simulink library "sm_car_lib"  (R2023a)
settings: Solver=VariableStepAuto  StartTime=0.0  StopTime=10.0  RelTol=1e-3
undefined symbols (not defined in the file or in its folder): Brakes, clr_upr, hp_la_out, hp_ua_out, opc_upr, radius_upr, rhs_hp, Steer, Z
libraries: Scene_Utilities x11, Suspension_Utilities x11, Vehicle_Inputs x5, Body_Utilities x3, World_Config_Utilities x2, Tire_Delft x2, Body_Axle1 x1, Body_Axle2 x1, Body_Axle3 x1, Brakes_Axle2_HydraulicValves_Channel4 x1, Brakes_Axle3_HydraulicValves_Channel6 x1, Brakes_Axle1_PedalAbstract_Disc x1
Description:
  | Simscape Vehicle Templates Library
  | 
  | Copyright 2018-2024 The MathWorks, Inc.
settings Model: Creator=mwalker  LastModifiedBy=smiller
settings SolverCC: AlgebraicLoopSolver=TrustRegion
settings DataIOCC: ReturnWorkspaceOutputs=off
settings DebuggingCC: UnconnectedInputMsg=warning  UnconnectedOutputMsg=warning  UnconnectedLineMsg=warning  ArithmeticOperatorsInVariantConditions=warning
settings ModelReferenceCC: EnableRefExpFcnMdlSchedulingChecks=on
settings SFSimCC: SimUseLocalCustomCode=off  CustomCodeUndefinedFunction=UseInterfaceOnly
settings RTWCC: RTWUseLocalCustomCode=off

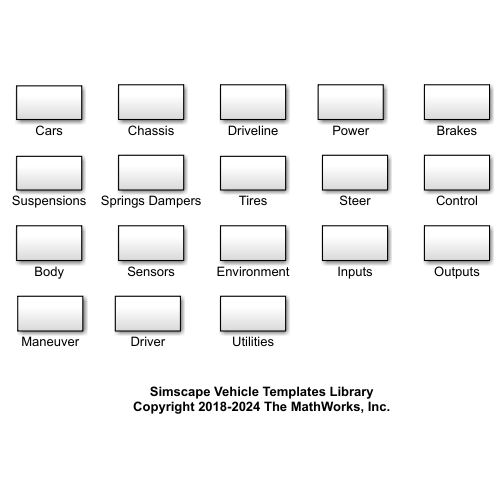
[thumbnail: Simulink's stored preview of the top-level diagram]
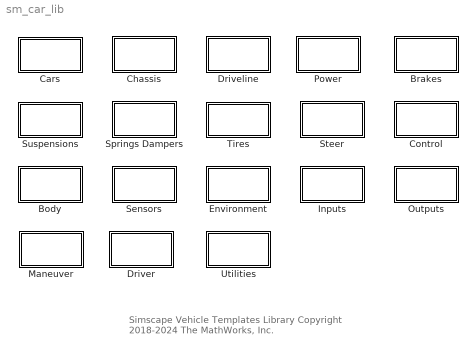
== system sm_car_lib ==
  note: Simscape Vehicle Templates Library
      | Copyright 2018-2024 The MathWorks, Inc.
  Body : Subsystem
  Brakes : Subsystem
  Cars : Subsystem
  Chassis : Subsystem
  Control : Subsystem
  Driveline : Subsystem
  Driver : Subsystem
  Environment : Subsystem
  Inputs : Subsystem
  Maneuver : Subsystem
  Outputs : Subsystem
  Power : Subsystem
  Sensors : Subsystem
  Springs Dampers : Subsystem
  Steer : Subsystem
  Suspensions : Subsystem
  Tires : Subsystem
  Utilities : Subsystem

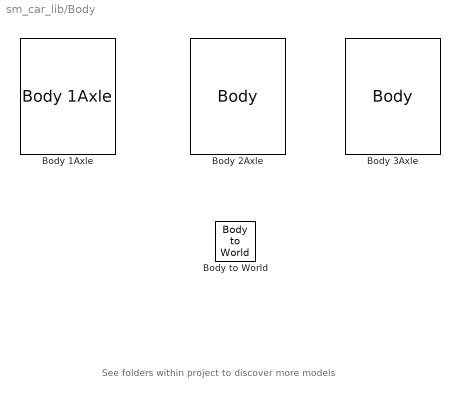
== system sm_car_lib/Body ==
  note: See folders within project to discover more models
  Body 1Axle : Body_Axle1/Body 1Axle  hp_mount_fa=Chassis.Body.sAxleF.Value  hp_mount_hitch=Chassis.Body.sAxleR.Value  hp_mount_power=Chassis.Body.sPower.Value  hp_chassis_cg=Chassis.Body.sCG.Value  chassis_mass=Chassis.Body.m.Value  chassis_inertia=Chassis.Body.J.Value  clr_chassis_hp_cg=Visual.hp.clr  opc_chassis_hp_cg=Visual.hp.opc  size_chassis_hp_cg=Visual.hp.rad  BodyGeometry=Chassis.Body.BodyGeometry
  Body 2Axle : Body_Axle2/Body  hp_mount_a1=Chassis.Body.sAxle1.Value  hp_mount_a2=Chassis.Body.sAxle2.Value  hp_mount_power=Vehicle.Chassis.Body.sPower.Value  hp_chassis_cg=Vehicle.Chassis.Body.sCG.Value  hp_mount_hitchf=Chassis.Body.sHitchF.Value  hp_mount_hitchr=Vehicle.Chassis.Body.sHitchR.Value  chassis_mass=Vehicle.Chassis.Body.m.Value  chassis_inertia=Vehicle.Chassis.Body.J.Value  clr_chassis_hp_cg=Visual.hp.clr  opc_chassis_hp_cg=Visual.hp.opc  size_chassis_hp_cg=Visual.hp.rad  BodyGeometry=Vehicle.Chassis.Body.BodyGeometry  Passenger=Vehicle.Chassis.Body.Passenger  BodyLoad=Body.BodyLoad
  Body 3Axle : Body_Axle3/Body  hp_mount_a1=Chassis.Body.sAxle1.Value  hp_mount_a2=Chassis.Body.sAxle2.Value  hp_mount_a3=Chassis.Body.sAxle3.Value  hp_mount_power=Vehicle.Chassis.Body.sPower.Value  hp_chassis_cg=Vehicle.Chassis.Body.sCG.Value  hp_mount_hitchf=Chassis.Body.sHitchF.Value  hp_mount_hitchr=Vehicle.Chassis.Body.sHitchR.Value  chassis_mass=Vehicle.Chassis.Body.m.Value  chassis_inertia=Vehicle.Chassis.Body.J.Value  clr_chassis_hp_cg=Visual.hp.clr  opc_chassis_hp_cg=Visual.hp.opc  size_chassis_hp_cg=Visual.hp.rad  BodyGeometry=Vehicle.Chassis.Body.BodyGeometry  Passenger=Vehicle.Chassis.Body.Passenger
  Body to World : Body_Utilities/Body to World  Init=Init.Chassis  SpecifyPosTarget=on

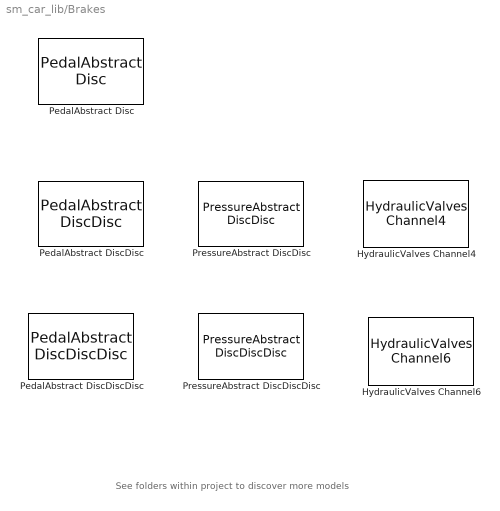
== system sm_car_lib/Brakes ==
  note: See folders within project to discover more models
  HydraulicValves Channel4 : Brakes_Axle2_HydraulicValves_Channel4/HydraulicValves Channel4  Tag=PublishSubsystem  VariantControl=HydraulicValves_Channel4  d_caliper_bore_a1=Brakes.Axle1.Caliper.lCylinderDiameter.Value  d_caliper_bore_a2=Brakes.Axle2.Caliper.lCylinderDiameter.Value  brk_pad_rad_a1=Brakes.Axle1.DiscAndPad.lMeanRadius.Value  brk_pad_rad_a2=Brakes.Axle2.DiscAndPad.lMeanRadius.Value  brk_cyl_bore_a1=Brakes.Axle1.Caliper.lCylinderDiameter.Value  brk_cyl_bore_a2=Brakes.Axle2.Caliper.lCylinderDiameter.Value  brk_n_pads_a1=Brakes.Axle1.DiscAndPad.NPads.Value  brk_n_pads_a2=Brakes.Axle2.DiscAndPad.NPads.Value  brk_mu_static_a1=Brakes.Axle1.DiscAndPad.rMuStatic.Value  brk_mu_static_a2=Brakes.Axle2.DiscAndPad.rMuStatic.Value  brk_mu_kin_a1=Brakes.Axle1.DiscAndPad.rMuKinetic.Value  brk_mu_kin_a2=Brakes.Axle2.DiscAndPad.rMuKinetic.Value  brk_trans_vel_a1=Brakes.Axle1.DiscAndPad.nTransition.Value  brk_trans_vel_a2=Brakes.Axle2.DiscAndPad.nTransition.Value  brk_visc_coef_a1=Brakes.Axle1.DiscAndPad.dViscous.Value  brk_visc_coef_a2=Brakes.Axle2.DiscAndPad.dViscous.Value  spr_rate=Brakes.Axle1.ValveApply.kSpring.Value  D=Brakes.Axle1.ValveApply.bDamper.Value  area_max_apply=Brakes.Axle1.ValveApply.AMax.Value  open_max_apply=Brakes.Axle1.ValveApply.xMax.Value  area_max_rel=Brakes.Axle1.ValveRelease.AMax.Value  open_max_rel=Brakes.Axle1.ValveRelease.xMax.Value  p_max_a1=Brakes.Axle1.Caliper.pMax.Value  p_max_a2=Brakes.Axle2.Caliper.pMax.Value  brkTs=Brakes.Axle1.ValveApply.fValveTime.Value
  HydraulicValves Channel6 : Brakes_Axle3_HydraulicValves_Channel6/HydraulicValves Channel6  Tag=PublishSubsystem  VariantControl=HydraulicValves_Channel6  d_caliper_bore_a1=Brakes.Axle1.Caliper.lCylinderDiameter.Value  d_caliper_bore_a2=Brakes.Axle2.Caliper.lCylinderDiameter.Value  d_caliper_bore_a3=Brakes.Axle3.Caliper.lCylinderDiameter.Value  brk_pad_rad_a1=Brakes.Axle1.DiscAndPad.lMeanRadius.Value  brk_pad_rad_a2=Brakes.Axle2.DiscAndPad.lMeanRadius.Value  brk_pad_rad_a3=Brakes.Axle3.DiscAndPad.lMeanRadius.Value  brk_cyl_bore_a1=Brakes.Axle1.Caliper.lCylinderDiameter.Value  brk_cyl_bore_a2=Brakes.Axle2.Caliper.lCylinderDiameter.Value  brk_cyl_bore_a3=Brakes.Axle3.Caliper.lCylinderDiameter.Value  brk_n_pads_a1=Brakes.Axle1.DiscAndPad.NPads.Value  brk_n_pads_a2=Brakes.Axle2.DiscAndPad.NPads.Value  brk_n_pads_a3=Brakes.Axle3.DiscAndPad.NPads.Value  brk_mu_static_a1=Brakes.Axle1.DiscAndPad.rMuStatic.Value  brk_mu_static_a2=Brakes.Axle2.DiscAndPad.rMuStatic.Value  brk_mu_static_a3=Brakes.Axle3.DiscAndPad.rMuStatic.Value  brk_mu_kin_a1=Brakes.Axle1.DiscAndPad.rMuKinetic.Value  brk_mu_kin_a2=Brakes.Axle2.DiscAndPad.rMuKinetic.Value  brk_mu_kin_a3=Brakes.Axle3.DiscAndPad.rMuKinetic.Value  brk_trans_vel_a1=Brakes.Axle1.DiscAndPad.nTransition.Value  brk_trans_vel_a2=Brakes.Axle2.DiscAndPad.nTransition.Value  brk_trans_vel_a3=Brakes.Axle3.DiscAndPad.nTransition.Value  brk_visc_coef_a1=Brakes.Axle1.DiscAndPad.dViscous.Value  brk_visc_coef_a2=Brakes.Axle2.DiscAndPad.dViscous.Value  brk_visc_coef_a3=Brakes.Axle3.DiscAndPad.dViscous.Value  spr_rate=Brakes.Axle1.ValveApply.kSpring.Value  D=Brakes.Axle1.ValveApply.bDamper.Value  area_max_apply=Brakes.Axle1.ValveApply.AMax.Value  open_max_apply=Brakes.Axle1.ValveApply.xMax.Value  area_max_rel=Brakes.Axle1.ValveRelease.AMax.Value  open_max_rel=Brakes.Axle1.ValveRelease.xMax.Value  p_max_a1=Brakes.Axle1.Caliper.pMax.Value  p_max_a2=Brakes.Axle2.Caliper.pMax.Value  p_max_a3=Brakes.Axle3.Caliper.pMax.Value  brkTs=Brakes.Axle1.ValveApply.fValveTime.Value
  PedalAbstract Disc : Brakes_Axle1_PedalAbstract_Disc/PedalAbstract Disc  Tag=PublishSubsystem  VariantControl=PedalAbstract_Disc  brk_pad_rad_a1=Brakes.Axle1.DiscAndPad.lMeanRadius.Value  brk_cyl_bore_a1=Brakes.Axle1.Caliper.lCylinderDiameter.Value  brk_n_pads_a1=Brakes.Axle1.DiscAndPad.NPads.Value  brk_mu_static_a1=Brakes.Axle1.DiscAndPad.rMuStatic.Value  brk_mu_kin_a1=Brakes.Axle1.DiscAndPad.rMuKinetic.Value  brk_trans_vel_a1=Brakes.Axle1.DiscAndPad.nTransition.Value  brk_visc_coef_a1=Brakes.Axle1.DiscAndPad.dViscous.Value  brk_max_p_a1=Brakes.Axle1.Caliper.pMax.Value  brk_filt_a1=1/Brakes.Axle1.Caliper.fActuatorCutoff.Value
  PedalAbstract DiscDisc : Brakes_Axle2_PedalAbstract_DiscDisc/PedalAbstract DiscDisc  Tag=PublishSubsystem  VariantControl=PedalAbstract_DiscDisc  brk_pad_rad_a1=Brakes.Axle1.DiscAndPad.lMeanRadius.Value  brk_pad_rad_a2=Brakes.Axle2.DiscAndPad.lMeanRadius.Value  brk_cyl_bore_a1=Brakes.Axle1.Caliper.lCylinderDiameter.Value  brk_cyl_bore_a2=Brakes.Axle2.Caliper.lCylinderDiameter.Value  brk_n_pads_a1=Brakes.Axle1.DiscAndPad.NPads.Value  brk_n_pads_a2=Brakes.Axle2.DiscAndPad.NPads.Value  brk_mu_static_a1=Brakes.Axle1.DiscAndPad.rMuStatic.Value  brk_mu_static_a2=Brakes.Axle2.DiscAndPad.rMuStatic.Value  brk_mu_kin_a1=Brakes.Axle1.DiscAndPad.rMuKinetic.Value  brk_mu_kin_a2=Brakes.Axle2.DiscAndPad.rMuKinetic.Value  brk_trans_vel_a1=Brakes.Axle1.DiscAndPad.nTransition.Value  brk_trans_vel_a2=Brakes.Axle2.DiscAndPad.nTransition.Value  brk_visc_coef_a1=Brakes.Axle1.DiscAndPad.dViscous.Value  brk_visc_coef_a2=Brakes.Axle2.DiscAndPad.dViscous.Value  brk_max_p_a1=Brakes.Axle1.Caliper.pMax.Value  brk_max_p_a2=Brakes.Axle2.Caliper.pMax.Value  brk_filt_a1=1/Brakes.Axle1.Caliper.fActuatorCutoff.Value  brk_filt_a2=1/Brakes.Axle2.Caliper.fActuatorCutoff.Value
  PedalAbstract DiscDiscDisc : Brakes_Axle3_PedalAbstract_DiscDiscDisc/PedalAbstract DiscDiscDisc  Tag=PublishSubsystem  VariantControl=PedalAbstract_DiscDiscDisc  brk_pad_rad_a1=Brakes.Axle1.DiscAndPad.lMeanRadius.Value  brk_pad_rad_a2=Brakes.Axle2.DiscAndPad.lMeanRadius.Value  brk_pad_rad_a3=Brakes.Axle3.DiscAndPad.lMeanRadius.Value  brk_cyl_bore_a1=Brakes.Axle1.Caliper.lCylinderDiameter.Value  brk_cyl_bore_a2=Brakes.Axle2.Caliper.lCylinderDiameter.Value  brk_cyl_bore_a3=Brakes.Axle3.Caliper.lCylinderDiameter.Value  brk_n_pads_a1=Brakes.Axle1.DiscAndPad.NPads.Value  brk_n_pads_a2=Brakes.Axle2.DiscAndPad.NPads.Value  brk_n_pads_a3=Brakes.Axle3.DiscAndPad.NPads.Value  brk_mu_static_a1=Brakes.Axle1.DiscAndPad.rMuStatic.Value  brk_mu_static_a2=Brakes.Axle2.DiscAndPad.rMuStatic.Value  brk_mu_static_a3=Brakes.Axle3.DiscAndPad.rMuStatic.Value  brk_mu_kin_a1=Brakes.Axle1.DiscAndPad.rMuKinetic.Value  brk_mu_kin_a2=Brakes.Axle2.DiscAndPad.rMuKinetic.Value  brk_mu_kin_a3=Brakes.Axle3.DiscAndPad.rMuKinetic.Value  brk_trans_vel_a1=Brakes.Axle1.DiscAndPad.nTransition.Value  brk_trans_vel_a2=Brakes.Axle2.DiscAndPad.nTransition.Value  brk_trans_vel_a3=Brakes.Axle3.DiscAndPad.nTransition.Value  brk_visc_coef_a1=Brakes.Axle1.DiscAndPad.dViscous.Value  brk_visc_coef_a2=Brakes.Axle2.DiscAndPad.dViscous.Value  brk_visc_coef_a3=Brakes.Axle3.DiscAndPad.dViscous.Value  brk_max_p_a1=Brakes.Axle1.Caliper.pMax.Value  brk_max_p_a2=Brakes.Axle2.Caliper.pMax.Value  brk_max_p_a3=Brakes.Axle3.Caliper.pMax.Value  brk_filt_a1=1/Brakes.Axle1.Caliper.fActuatorCutoff.Value  brk_filt_a2=1/Brakes.Axle2.Caliper.fActuatorCutoff.Value  brk_filt_a3=1/Brakes.Axle3.Caliper.fActuatorCutoff.Value
  PressureAbstract DiscDisc : Brakes_Axle2_PressureAbstract_DiscDisc/PressureAbstract DiscDisc  Tag=PublishSubsystem  VariantControl=PressureAbstract_DiscDisc  brk_pad_rad_a1=Brakes.Axle1.DiscAndPad.lMeanRadius.Value  brk_pad_rad_a2=Brakes.Axle2.DiscAndPad.lMeanRadius.Value  brk_cyl_bore_a1=Brakes.Axle1.Caliper.lCylinderDiameter.Value  brk_cyl_bore_a2=Brakes.Axle2.Caliper.lCylinderDiameter.Value  brk_n_pads_a1=Brakes.Axle1.DiscAndPad.NPads.Value  brk_n_pads_a2=Brakes.Axle2.DiscAndPad.NPads.Value  brk_mu_static_a1=Brakes.Axle1.DiscAndPad.rMuStatic.Value  brk_mu_static_a2=Brakes.Axle2.DiscAndPad.rMuStatic.Value  brk_mu_kin_a1=Brakes.Axle1.DiscAndPad.rMuKinetic.Value  brk_mu_kin_a2=Brakes.Axle2.DiscAndPad.rMuKinetic.Value  brk_trans_vel_a1=Brakes.Axle1.DiscAndPad.nTransition.Value  brk_trans_vel_a2=Brakes.Axle2.DiscAndPad.nTransition.Value  brk_visc_coef_a1=Brakes.Axle1.DiscAndPad.dViscous.Value  brk_visc_coef_a2=Brakes.Axle2.DiscAndPad.dViscous.Value  brk_filt_a1=1/Brakes.Axle1.Caliper.fActuatorCutoff.Value  brk_filt_a2=1/Brakes.Axle2.Caliper.fActuatorCutoff.Value
  PressureAbstract DiscDiscDisc : Brakes_Axle3_PressureAbstract_DiscDiscDisc/PressureAbstract DiscDiscDisc  Tag=PublishSubsystem  VariantControl=PressureAbstract_DiscDiscDisc  brk_pad_rad_a1=Brakes.Axle1.DiscAndPad.lMeanRadius.Value  brk_pad_rad_a2=Brakes.Axle2.DiscAndPad.lMeanRadius.Value  brk_pad_rad_a3=Brakes.Axle3.DiscAndPad.lMeanRadius.Value  brk_cyl_bore_a1=Brakes.Axle1.Caliper.lCylinderDiameter.Value  brk_cyl_bore_a2=Brakes.Axle2.Caliper.lCylinderDiameter.Value  brk_cyl_bore_a3=Brakes.Axle3.Caliper.lCylinderDiameter.Value  brk_n_pads_a1=Brakes.Axle1.DiscAndPad.NPads.Value  brk_n_pads_a2=Brakes.Axle2.DiscAndPad.NPads.Value  brk_n_pads_a3=Brakes.Axle3.DiscAndPad.NPads.Value  brk_mu_static_a1=Brakes.Axle1.DiscAndPad.rMuStatic.Value  brk_mu_static_a2=Brakes.Axle2.DiscAndPad.rMuStatic.Value  brk_mu_static_a3=Brakes.Axle3.DiscAndPad.rMuStatic.Value  brk_mu_kin_a1=Brakes.Axle1.DiscAndPad.rMuKinetic.Value  brk_mu_kin_a2=Brakes.Axle2.DiscAndPad.rMuKinetic.Value  brk_mu_kin_a3=Brakes.Axle3.DiscAndPad.rMuKinetic.Value  brk_trans_vel_a1=Brakes.Axle1.DiscAndPad.nTransition.Value  brk_trans_vel_a2=Brakes.Axle2.DiscAndPad.nTransition.Value  brk_trans_vel_a3=Brakes.Axle3.DiscAndPad.nTransition.Value  brk_visc_coef_a1=Brakes.Axle1.DiscAndPad.dViscous.Value  brk_visc_coef_a2=Brakes.Axle2.DiscAndPad.dViscous.Value  brk_visc_coef_a3=Brakes.Axle3.DiscAndPad.dViscous.Value  brk_filt_a1=1/Brakes.Axle1.Caliper.fActuatorCutoff.Value  brk_filt_a2=1/Brakes.Axle2.Caliper.fActuatorCutoff.Value  brk_filt_a3=1/Brakes.Axle3.Caliper.fActuatorCutoff.Value

== system sm_car_lib/Cars ==
  note: See folders within project to discover more models
  Vehicle Axle1 : Vehicle_Axle1/Vehicle 1Axle  Tag=PublishSubsystem  VariantControl=NS_Con  Vehicle=Trailer  Init=Init  veh_index=61
  Vehicle Axle2 : Vehicle_Axle2/Vehicle  Tag=PublishSubsystem  VariantControl=NS_Con  Vehicle=Vehicle  Init=Init  SpecifyPosTarget=on  veh_index=1  mask_image_name=sm_car_vehicle_hamba_IMAGE.png
  Vehicle Axle3 : Vehicle_Axle3/Vehicle  Tag=PublishSubsystem  VariantControl=NS_Con  Vehicle=Vehicle  Init=Init  veh_index=1  mask_image_name=sm_car_vehicle_hambalg_IMAGE.png

== system sm_car_lib/Chassis ==
  note: See folders within project to discover more models
  Chassis Axle1 : Chassis_Axle1/Chassis  Tag=PublishSubsystem  VariantControl=Chassis  Chassis=Vehicle.Chassis  Init=Init  veh_index=61
  Chassis Axle2 : Chassis_Axle2/Chassis  Tag=PublishSubsystem  VariantControl=Chassis  Chassis=Vehicle.Chassis  Init=Init  mask_image_name=sm_car_vehicle_chassis_custom_IMAGE.png  veh_index=1
  Chassis Axle3 : Chassis_Axle3/Chassis  Tag=PublishSubsystem  VariantControl=Chassis  Chassis=Vehicle.Chassis  Init=Init  mask_image_name=sm_car_vehicle_chassis_custom_IMAGE.png  veh_index=1

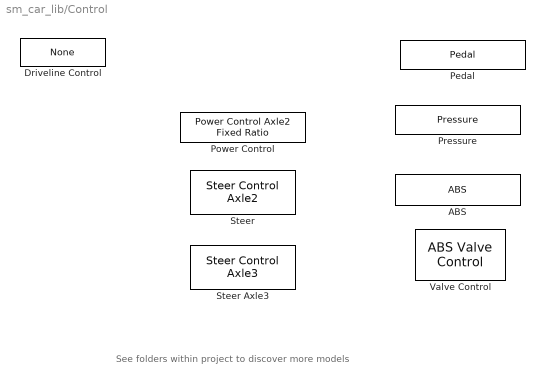
== system sm_car_lib/Control ==
  note: See folders within project to discover more models
  ABS : Brake_Control_ABS/ABS  VariantControl=ABS  abs_tire_radiusF=abs_tire_radiusF  abs_tire_radiusR=abs_tire_radiusR
  Driveline Control : Driveline_Control_Axle2_None/None  SystemSampleTime=-1  VariantActivationTime=update diagram  Latency=0  AutoFrameSizeCalculation=off
  Pedal : Brake_Control_Pedal/Pedal  SystemSampleTime=-1  VariantControl=Pedal  VariantActivationTime=update diagram  Latency=0  AutoFrameSizeCalculation=off
  Power Control : Power_Control_Axle2_FixedRatio/Power Control Axle2 Fixed Ratio  trq_max=1600  trq_ratio_front=1  trq_rate_up=300  trq_rate_down=-5000
  Pressure : Brake_Control_Pressure/Pressure  SystemSampleTime=-1  VariantControl=Pressure  VariantActivationTime=update diagram  Latency=0  AutoFrameSizeCalculation=off
  Steer : Steer_Control_Axle2/Steer Control Axle2  Steer=Control.Default.Steer
  Steer Axle3 : Steer_Control_Axle3/Steer Control Axle3  nSteerA2=Control.Default.steer_ratio_axle2  nSteerA3=Control.Default.steer_ratio_axle3
  Valve Control : Brake_Control_ABS_Valve/ABS Valve Control  SystemSampleTime=-1  VariantActivationTime=update diagram  Latency=0  AutoFrameSizeCalculation=off

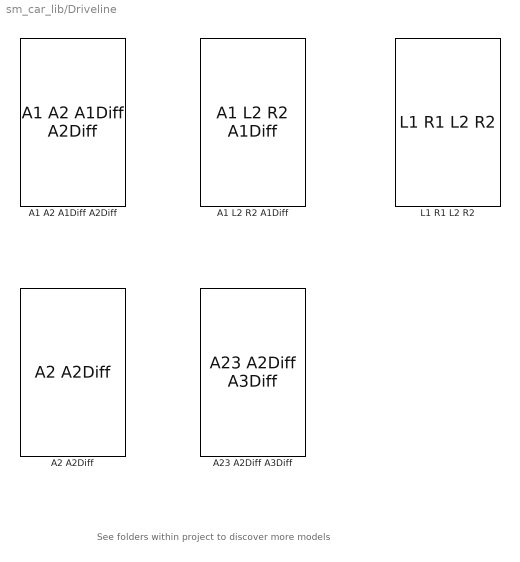
== system sm_car_lib/Driveline ==
  note: See folders within project to discover more models
  A1 A2 A1Diff A2Diff : Driveline_Axle2_A1_A2_A1Diff_A2Diff/A1 A2 A1Diff A2Diff  Tag=PublishSubsystem  VariantControl=A1_A2_A1Diff_A2Diff
  A1 L2 R2 A1Diff : Driveline_Axle2_A1_L2_R2_A1Diff/A1 L2 R2 A1Diff  Tag=PublishSubsystem  VariantControl=A1_L2_R2_A1Diff
  A2 A2Diff : Driveline_Axle3_A2_A2Diff/A2 A2Diff  Tag=PublishSubsystem  VariantControl=A2_A2Diff
  A23 A2Diff A3Diff : Driveline_Axle3_A23_A2Diff_A3Diff/A23 A2Diff A3Diff  Tag=PublishSubsystem  VariantControl=A23_A2Diff_A3Diff
  L1 R1 L2 R2 : Driveline_Axle2_L1_R1_L2_R2/L1 R1 L2 R2  Tag=PublishSubsystem  VariantControl=L1_R1_L2_R2

== system sm_car_lib/Driver ==
  note: See folders within project to discover more models
  Long Lat Stanley : Driver_Long_Lateral/Driver  Driver=Driver
  Open Loop : Driver_Open_Loop/Open Loop  Maneuver=Maneuver

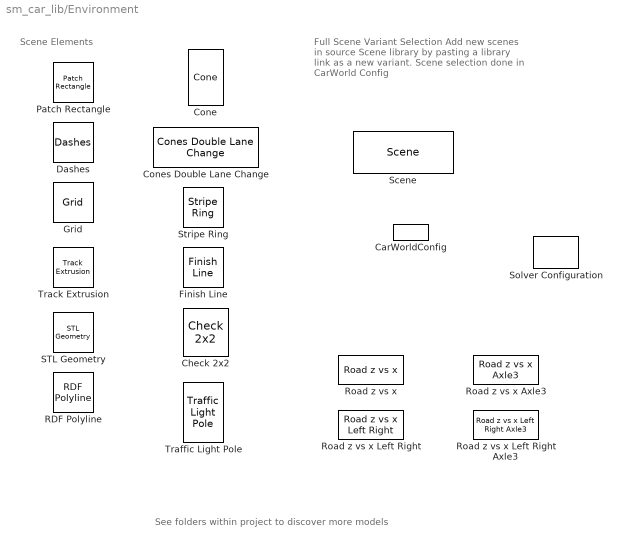
== system sm_car_lib/Environment ==
  note: Full Scene Variant Selection
      | Add new scenes in source
      | Scene library by pasting a library
      | link as a new variant.
      | Scene selection done
      | in CarWorld Config
  note: Scene Elements
  note: See folders within project to discover more models
  CarWorldConfig : World_Config_Utilities/CarWorldConfig  UseLocalSolver=off  LocalSolverChoice=Backward Euler  LocalSolverSampleTime=0.005  DoFixedCost=off  MaxNonlinIter=3  popup_scene=Plane Grid  popup_gravity=Constant  GravityVector=[0 0 -9.80665]
      settings: AttributesFormatString=|
      | %<popup_scene>
      | Local Solver: %<UseLocalSolver>
  Check 2x2 : Scene_Utilities/Check 2x2  square_lwh=[0.01 1 1]
  Cone : Scene_Utilities/Cone  height=1  baseThickness=0.1  baseWidth=0.6  coneBaseDiameter=0.4  coneTopDiameter=0.1  reflectiveStripHeight=0.5  coneColor=[1 0.6 0]  reflectiveStripColor=[0.75 0.75 0.75]
  Cones Double Lane Change : Scene_Utilities/Cones Double Lane Change  lane_width=3.3  lane_separation=4.1  start_lane_a=173.8  A1_to_A5=12.5  A_to_B_x=12.7  B1_to_B5=12.3  B_to_C_x=12.7  C1_to_C5=12  height=0.6  baseThickness=0.04  baseWidth=0.5  coneBaseDiameter=0.24  coneTopDiameter=0.06  reflectiveStripHeight=0.3  coneColor=[248 78 25]/255  reflectiveStripColor=[0.75 0.75 0.75]
  Dashes : Scene_Utilities/Dashes  dash_pitch=7.5  num_dashes=4  dash_l=3  dash_h=2  dash_w=0.15  thickness_base=4  dash_clr=[1 1 1]  dash_opc=1
  Finish Line : Scene_Utilities/Finish Line  post_h=6  post_r=0.5  line_w=18  post_clr=[0.8 0.0 0.2]  post_opc=1  offset_xyz=[0 0 0]  offset_yaw=0  offset_pitch=0  offset_roll=0
  Grid : Scene_Utilities/Grid  grid_x=400  grid_y=400  grid_z=0.02  grid_line_width=0.08  grid_num_sq_x=10  grid_num_sq_y=17  grid_clr=[1 1 1]  grid_opc=1
  Patch Rectangle : Scene_Utilities/Patch Rectangle  gp_l=400  gp_w=400  gp_h=0.01  gp_clr=[0.8000 0.8000 0.8000]  gp_opc=1
  RDF Polyline : Scene_Utilities/RDF Polyline  road_extr_data_L=RDF_Rough_Road.Road.extr_data_L  road_extr_data_R=RDF_Rough_Road.Road.extr_data_R  road_profile_sep=RDF_Rough_Road.Road.profile_separation  road_w=RDF_Rough_Road.Road.w  road_x=RDF_Rough_Road.Road.x  road_z=RDF_Rough_Road.Road.z  road_yaw=RDF_Rough_Road.Road.yaw  road_clr=RDF_Rough_Road.Road.clr  road_opc=RDF_Rough_Road.Road.opc
  Road z vs x Left Right : Surface_Profile_Axle2_zx_LR/Road z vs x Left Right  VariantControl=Variant  dist_x_l=flipud(Scene.RDF_Plateau.Road.extr_data_L(45:end,1))  height_z_l=flipud(Scene.RDF_Plateau.Road.extr_data_L(45:end,2))  dist_x_r=flipud(Scene.RDF_Plateau.Road.extr_data_R(45:end,1))  height_z_r=flipud(Scene.RDF_Plateau.Road.extr_data_R(45:end,2))
  Road z vs x Left Right Axle3 : Surface_Profile_Axle3_zx_LR/Road z vs x Left Right Axle3  VariantControl=Variant  dist_x_l=flipud(Scene.RDF_Plateau.Road.extr_data_L(45:end,1))  height_z_l=flipud(Scene.RDF_Plateau.Road.extr_data_L(45:end,2))  dist_x_r=flipud(Scene.RDF_Plateau.Road.extr_data_R(45:end,1))  height_z_r=flipud(Scene.RDF_Plateau.Road.extr_data_R(45:end,2))
  "Road z vs x " : Surface_Profile_Axle2_zx/Road z vs x   VariantControl=Variant  dist_x=flipud(Scene.RDF_Plateau.Road.extr_data_L(45:end,1))  height_z=flipud(Scene.RDF_Plateau.Road.extr_data_L(45:end,2))
  Road z vs x Axle3 : Surface_Profile_Axle3_zx/Road z vs x Axle3  VariantControl=Variant  dist_x=flipud(Scene.RDF_Plateau.Road.extr_data_L(45:end,1))  height_z=flipud(Scene.RDF_Plateau.Road.extr_data_L(45:end,2))
  STL Geometry : Scene_Utilities/STL Geometry  stl_file='Bar1_Default_sldprt.STL'  stl_units='m'  stl_clr=[0.8000 0.8000 0.8000]  stl_opc=1  stl_x=0  stl_y=0  stl_z=0  stl_yaw=0  stl_pitch=0  stl_roll=0
  Scene : Scene_Systems/Scene  SystemSampleTime=-1  LabelModeActiveChoice=Road_Two_Lane  VariantActivationTime=update diagram  Latency=0  AutoFrameSizeCalculation=off
      settings: AttributesFormatString=%<LabelModeActiveChoice>
  Solver Configuration : nesl_utility/Solver Configuration  PhysicalDomain=network_engine_domain  SubClassName=solver  LeftPortType=input  RightPortType=generic  Tones=[]  Harmonics=[]  SimulateNoise=off  Profile=off  UseLocalSampling=off  EnableSwitchedLinearOptims=on  FrequencyDomain=off  UseCCode=off  RelTol=0.001  AbsTol=1e-06  MinStep=1e-09  ToWorkspace=off  RevertToSquareIcSolve=off  NumHomotopyIterations=100  PhasorMode=off  PhasorModeNumHarmonics=1  IndexReductionMethod=DerivativeReplacement  DoDC=off  ResidualTolerance=1e-09  UseLocalSolver=on  LocalSolverChoice=NE_BACKWARD_EULER_ADVANCER  LocalSolverSampleTime=0.001  DoFixedCost=on  MaxNonlinIter=3  MaxModeIter=2  ComputeImpulses=off  ImpulseIterations=2  LinearAlgebra=auto  LinearAlgebraNumThread=0  EquationFormulation=NE_TIME_EF  DelaysMemoryBudget=1024  AutomaticFiltering=on  FilteringTimeConstant=0.001  PartitionStorageMethod=AS_NEEDED  PartitionMemoryBudget=1024  PartitionMethod=FAST
  Stripe Ring : Scene_Utilities/Stripe Ring  circ_d=circ_out.d  circ_a1=circ_out.ang1  circ_a2=circ_out.ang2  circ_w=circ_out.w  circ_h=circ_out.h  circ_clr=circ_out.clr  circ_opc=circ_out.opc
  Track Extrusion : Scene_Utilities/Track Extrusion  track_ctrline=[sin(0:0.1:(2*pi-0.1))' cos(0:0.1:(2*pi-0.1))' cos(0:0.1:(2*pi-0.1))']*10  track_w=2  track_h=0.1  track_x=0  track_y=0  track_z=0  track_yaw=0  track_clr=[0.8000 0.8000 0.8000]  track_opc=1
  Traffic Light Pole : Object_Traffic_Light/Traffic Light Pole  clr_tlp_housing=[0.5 0.5 0.5]  offset_tlp=[0 258 2]  orient_tlp=pi*1.1  pole_height_tlp=2

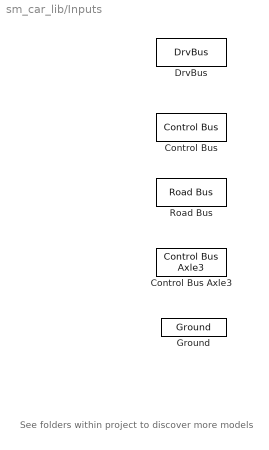
== system sm_car_lib/Inputs ==
  note: See folders within project to discover more models
  Control Bus : Vehicle_Inputs/Control Bus  SystemSampleTime=-1  VariantActivationTime=update diagram  Latency=0  AutoFrameSizeCalculation=off
  Control Bus Axle3 : Vehicle_Inputs/Control Bus Axle3  SystemSampleTime=-1  VariantActivationTime=update diagram  Latency=0  AutoFrameSizeCalculation=off
  DrvBus : Vehicle_Inputs/DrvBus  SystemSampleTime=-1  VariantActivationTime=update diagram  Latency=0  AutoFrameSizeCalculation=off
  Ground : Vehicle_Inputs/Ground  SystemSampleTime=-1  VariantActivationTime=update diagram  Latency=0  AutoFrameSizeCalculation=off
  Road Bus : Vehicle_Inputs/Road Bus  SystemSampleTime=-1  VariantActivationTime=update diagram  Latency=0  AutoFrameSizeCalculation=off

== system sm_car_lib/Maneuver ==
  note: See folders within project to discover more models
  Check : World_Config_Utilities/Check  stop_speed=0.1  start_check_time=5  max_speed=0.4  start_check_time_max_speed=20000  lat_dev_threshold=8  start_check_time_ld=10000  start_check_time_end_lap=10000
  Maneuver : Maneuver_Get_Pose/Maneuver  Maneuver=Maneuver  popup_window=No

== system sm_car_lib/Outputs ==
  note: See folders within project to discover more models
  Terminator : Terminator
  VehBus : Vehicle_Outputs/VehBus  SystemSampleTime=-1  VariantActivationTime=update diagram  Latency=0  AutoFrameSizeCalculation=off
  wires:
  VehBus/1 -> Terminator/1

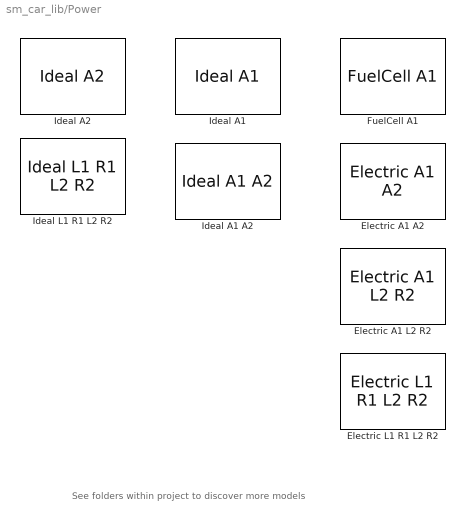
== system sm_car_lib/Power ==
  note: See folders within project to discover more models
  Electric A1 A2 : Power_Shaft2_Electric_A1_A2/Electric A1 A2  VariantControl=Electric_A1_A2  Power=Powertrain.Power
  Electric A1 L2 R2 : Power_Shaft3_Electric_A1_L2_R2/Electric A1 L2 R2  VariantControl=Electric_A1_L2_R2  Power=Powertrain.Power
  Electric L1 R1 L2 R2 : Power_Shaft4_Electric_L1_R1_L2_R2/Electric L1 R1 L2 R2  VariantControl=Electric_L1_R1_L2_R2  Power=Powertrain.Power
  FuelCell A1 : Power_Shaft1_FuelCell_A1/FuelCell A1  VariantControl=FuelCell_A1  Power=Powertrain.Power
  Ideal A1 : Power_Shaft1_Ideal_A1/Ideal A1  VariantControl=Ideal_A1  motor_ts_f=Power.ActuatorCutoffA1.Value
  Ideal A1 A2 : Power_Shaft2_Ideal_A1_A2/Ideal A1 A2  VariantControl=Ideal_A1_A2  motor_ts_a1=Power.ActuatorCutoffA1.Value  motor_ts_a2=Power.ActuatorCutoffA2.Value
  Ideal A2 : Power_Shaft1_Ideal_A2/Ideal A2  VariantControl=Ideal_A2  motor_ts_f=Power.ActuatorCutoffA2.Value
  Ideal L1 R1 L2 R2 : Power_Shaft4_Ideal_L1_R1_L2_R2/Ideal L1 R1 L2 R2  VariantControl=Ideal_L1_R1_L2_R2  motor_ts_l1=100  motor_ts_r1=100  motor_ts_l2=100  motor_ts_r2=100

== system sm_car_lib/Sensors ==
  note: See folders within project to discover more models
  Body Sensor : Body_Utilities/Body Sensor  offset_body_sensor=Vehicle.Chassis.Body.sCG.Value
  Body Sensor Empty : Body_Utilities/Body Sensor Empty  offset_body_sensor=Vehicle.Chassis.Body.sCG.Value

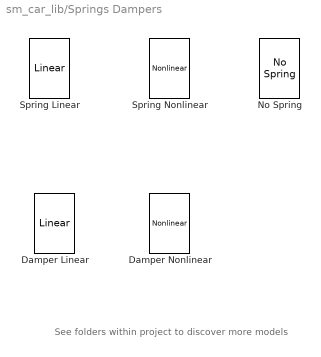
== system sm_car_lib/Springs Dampers ==
  note: See folders within project to discover more models
  Damper Linear : Damper_Linear/Linear  VariantControl=Linear  dam_b=Damper.Damping.d.Value  hp_dpr_top=Damper.Damping.sTop.Value  hp_dpr_bot=Damper.Damping.sBottom.Value  bs_lim_upper=Damper.Endstop.xMax.Value  bs_lim_lower=Damper.Endstop.xMin.Value  bs_k_upper=Damper.Endstop.KxMax.Value  bs_k_lower=Damper.Endstop.KxMin.Value  bs_b_upper=Damper.Endstop.dxMax.Value  bs_b_lower=Damper.Endstop.dxMin.Value  bs_region=Damper.Endstop.xTransition.Value
  Damper Nonlinear : Damper_Nonlinear/Nonlinear  VariantControl=Nonlinear  velocity_vector=Damper.Damping.vDamper.Value  force_vector=Damper.Damping.fDamper.Value  hp_dpr_top=Damper.Damping.sTop.Value  hp_dpr_bot=Damper.Damping.sBottom.Value  bs_lim_upper=Damper.Endstop.xMax.Value  bs_lim_lower=Damper.Endstop.xMin.Value  bs_k_upper=Damper.Endstop.KxMax.Value  bs_k_lower=Damper.Endstop.KxMin.Value  bs_b_upper=Damper.Endstop.dxMax.Value  bs_b_lower=Damper.Endstop.dxMin.Value  bs_region=Damper.Endstop.xTransition.Value
  No Spring : Spring_None/No Spring  VariantControl=No_Spring
  Spring Linear : Spring_Linear/Linear  VariantControl=Linear  spr_def0=Spring.xPreload.Value  spr_k=Spring.K.Value  spr_hp_top=Spring.sTop.Value  spr_hp_bot=Spring.sBottom.Value
  Spring Nonlinear : Spring_Nonlinear/Nonlinear  VariantControl=Nonlinear  spr_def0=Spring.xPreload.Value  deformation_vector=Spring.xSpring.Value  force_vector=Spring.fSpring.Value  spr_hp_top=Spring.sTop.Value  spr_hp_bot=Spring.sBottom.Value

== system sm_car_lib/Steer ==
  note: See folders within project to discover more models
  Rack : Steer_Rack_Only/Rack  Tag=PublishSubsystem  VariantControl=Rack  hp_mt_rack=Steer.Rack.sMount.Value  hp_out_rack=Steer.Rack.sOutboard.Value  rack_mass=Steer.Rack.m.Value  whl2rack_whlangle=Steer.Ratio_Table.aWheel.Value  whl2rack_rackdisp=Steer.Ratio_Table.xRack.Value  whl2rack_filter=1/Steer.Rack.fActuatorCutoff.Value  clr_rack=Visual.SteeringRack.clr  opc_rack=Visual.part.opc  radius_rack=Visual.SteeringRack.rad  clr_connhp=Visual.hp.clr  opc_connhp=Visual.hp.opc  size_connhp=Visual.hp.rad
  Rack Wheel : Steer_Rack_Wheel/Rack Wheel  Tag=PublishSubsystem  VariantControl=RackWheel  hp_wheel=Steer.Wheel.sMount.Value  wheel_axis_incl=Steer.Wheel.aAxis.Value  hp_mt_rack=Steer.Rack.sMount.Value  hp_out_rack=Steer.Rack.sOutboard.Value  Wheel=Steer.Wheel  rack_mass=Steer.Rack.m.Value  whl2rack_whlangle=Steer.Ratio_Table.aWheel.Value  whl2rack_rackdisp=Steer.Ratio_Table.xRack.Value  whl2rack_filter=1/Steer.Rack.fActuatorCutoff.Value  clr_rack=Visual.SteeringRack.clr  opc_rack=Visual.part.opc  radius_rack=Visual.SteeringRack.rad  clr_connhp=Visual.hp.clr  opc_connhp=Visual.hp.opc  size_connhp=Visual.hp.rad  clr_wheel=Visual.SteeringWheel.clr  opc_wheel=Visual.part.opc  DriverHuman=Steer.DriverHuman
  Wheel Driven Rack 1UJoint : Steer_Rack_WheelDrivenRack1UJoint/Wheel Driven Rack 1UJoint  Tag=PublishSubsystem  VariantControl=WheelDrivenRack1UJoint  hp_wheel=Steer.Wheel.sMount.Value  wheel_axis_incl=Steer.Wheel.aAxis.Value  hp_mt_rack=Steer.Rack.sMount.Value  hp_out_rack=Steer.Rack.sOutboard.Value  hp_pinion=Steer.Pinion.sMount.Value  Wheel=Steer.Wheel  len_sha_u=Steer.Shaft_Upper.xLength.Value  sha_u_mass=Steer.Shaft_Upper.m.Value  sha_l_mass=Steer.Shaft_Lower.m.Value  rad_pinion=Steer.Pinion.xRad.Value  pinion_mass=Steer.Pinion.m.Value  rack_mass=Steer.Rack.m.Value  whl2steer_filter=1/Steer.Rack.fActuatorCutoff.Value  clr_rack=Visual.SteeringRack.clr  opc_rack=Visual.part.opc  radius_rack=Visual.SteeringRack.rad  clr_shaft=Visual.SteeringShafts.clr  opc_shaft=Visual.part.opc  size_shaft=Visual.SteeringShafts.rad  clr_pinion=Visual.SteeringPinion.clr  opc_pinion=Visual.part.opc  len_pinion=Visual.SteeringPinion.len  clr_connhp=Visual.hp.clr  opc_connhp=Visual.hp.opc  size_connhp=Visual.hp.rad  clr_wheel=Visual.SteeringWheel.clr  opc_wheel=Visual.part.opc  DriverHuman=Steer.DriverHuman

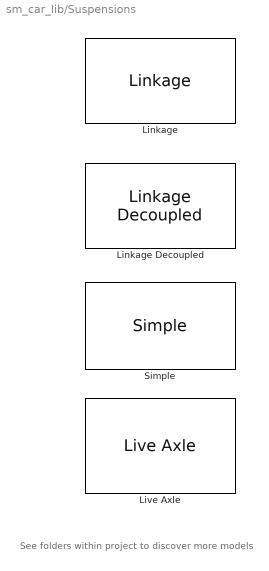
== system sm_car_lib/Suspensions ==
  note: See folders within project to discover more models
  Linkage : Suspension_Linkage/Linkage  VariantControl=Linkage
  Linkage Decoupled : Suspension_Linkage_Decoupled/Linkage Decoupled  VariantControl=Decoupled
  Live Axle : Suspension/Suspension and Steering/Live Axle  VariantControl=LiveAxle  LiveAxle=Susp.LiveAxle
  Simple : Susp_DOF15/Simple  VariantControl=Simple

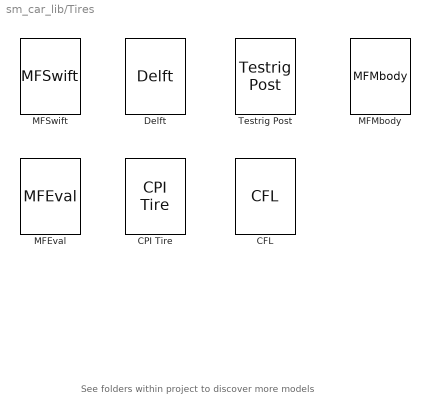
== system sm_car_lib/Tires ==
  note: See folders within project to discover more models
  CFL : Tire_CFL/CFL  VariantControl=CFL  popup_leftRight=Right  tire_radius=Tire.tire_radius.Value  rim_radius=Tire.rim_radius.Value  tire_width=Tire.tire_width.Value  rim_width=Tire.rim_width.Value  tyre_mass=Tire.tire_mass.Value  rim_mass=Tire.rim_mass.Value  tire_inertia=Tire.tire_J.Value  rim_inertia=Tire.rim_J.Value  plane_l=Tire.plane.l.Value  plane_w=Tire.plane.w.Value  k_contact=Tire.k.Value  b_contact=Tire.b.Value  mu_kinetic=Tire.mu_k.Value  mu_static=Tire.mu_s.Value  v_thr=Tire.v_thr.Value  TireBody=Tire.TireBody  clr_tyre_cfl=Visual.Tire.clr  opc_tyre_cfl=Visual.Tire.opc  clr_rim_cfl=Visual.Rim.clr  opc_rim_cfl=Visual.Rim.opc
  CPI Tire : Tire_Delft/CPI Tire  VariantControl=CPI  idtyre=0
  Delft : Tire_Delft/Delft  VariantControl=Delft  idtyre=tir_index  rim_inertia=Tire.mjRim.Value  tir_name=Tire.tirFile.Value  rdf_name=Tire.roadFile.Value  tire_side_mode=(2xxx) right  tire_contact=Tire.Contact.Value  tire_dynamics=Tire.Dynamics.Value  tire_slip=Tire.Slip.Value  TireBody=Tire.TireBody  popup_leftRight=Right  clr_tyre=Visual.Tire.clr  opc_tyre=Visual.Tire.opc  clr_rim=Visual.Rim.clr  opc_rim=Visual.Rim.opc
  MFEval : Tire_MFEval/MFEval  VariantControl=MFEval  tir_file=Tire.tirFile.Value  tir_side=2 right  tir_dynamics=Tire.Dynamics.Value  tir_mode=Tire.Slip.Value  TireBody=Tire.TireBody  popup_leftRight=Right  clr_tyre=Visual.Tire.clr  opc_tyre=Visual.Tire.opc  clr_rim=Visual.Rim.clr  opc_rim=Visual.Rim.opc
  MFMbody : Tire_MFMbody/MFMbody  VariantControl=MFMbody  tir_file=Tire.tirFile.Value  tire_side=Right  TireBody=Tire.TireBody  fcontactpatch=Tire.fContactPoint.Value  road_file=Tire.roadFile.Value  popup_leftRight=Right  clr_tyre=Visual.Tire.clr  opc_tyre=Visual.Tire.opc  clr_rim=Visual.Rim.clr  opc_rim=Visual.Rim.opc
  MFSwift : Tire_MFSwift/MFSwift  VariantControl=MFSwift  idtyre=tir_index  rim_inertia=Tire.mjRim.Value  tir_name=Tire.tirFile.Value  rdf_name=Tire.roadFile.Value  tire_side_mode=(x2xxx) right  tire_contact=Tire.Contact.Value  tire_dynamics=Tire.Dynamics.Value  tire_slip=Tire.Slip.Value  solver_enable=Tire.InternalSolver.Value  TireBody=Tire.TireBody  popup_leftRight=Right  clr_tyre=Visual.Tire.clr  opc_tyre=Visual.Tire.opc  clr_rim=Visual.Rim.clr  opc_rim=Visual.Rim.opc
  Testrig Post : Tire_Testrig_Post/Testrig Post  VariantControl=Testrig_Post  popup_leftRight=Right  tire_k=Tire.K.Value  tire_b=Tire.b.Value  tire_radius=Tire.tire_radius.Value  rim_radius=Tire.rim_radius.Value  tire_width=Tire.tire_width.Value  rim_width=Tire.rim_width.Value  tyre_mass=Tire.tire_mass.Value  rim_mass=Tire.rim_mass.Value  tire_inertia=Tire.tire_J.Value  rim_inertia=Tire.rim_J.Value  TireBody=Tire.TireBody  platform=Scene.Testrig_Post

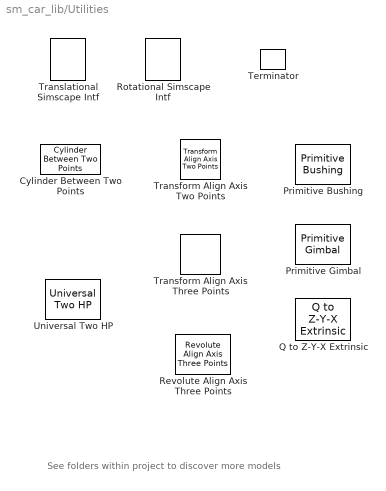
== system sm_car_lib/Utilities ==
  note: See folders within project to discover more models
  Cylinder Between Two Points : Suspension_Utilities/Cylinder Between Two Points  hp_b=hp_la_out.*rhs_hp  hp_f=hp_ua_out.*rhs_hp  Mass=0  clr_solid=clr_upr*0+[0.2 0.4 0.6]  opc_solid=opc_upr*0.5  rad_solid=radius_upr*1.5
  Primitive Bushing : Suspension_Utilities/Primitive Bushing  SystemSampleTime=-1  VariantActivationTime=update diagram  Latency=0  AutoFrameSizeCalculation=off
  Primitive Gimbal : Suspension_Utilities/Primitive Gimbal  SystemSampleTime=-1  VariantActivationTime=update diagram  Latency=0  AutoFrameSizeCalculation=off
  Q to Z-Y-X Extrinsic : Suspension_Utilities/Q to Z-Y-X Extrinsic  SystemSampleTime=-1  VariantActivationTime=update diagram  Latency=0  AutoFrameSizeCalculation=off
  Revolute Align Axis Three Points : Suspension_Utilities/Revolute Align Axis Three Points  popup_leftRight=Left  hp_1=[0 0 0]  hp_2=[1 0 1]  hp_3=[0 1 1]
  Rotational Simscape Intf : Suspension_Utilities/Rotational Simscape Intf  SystemSampleTime=-1  VariantActivationTime=update diagram  Latency=0  AutoFrameSizeCalculation=off
  Terminator : Suspension_Utilities/Terminator  SystemSampleTime=-1  VariantActivationTime=update diagram  Latency=0  AutoFrameSizeCalculation=off
  Transform Align Axis Three Points : Suspension_Utilities/Transform Align Axis Three Points  pt1=hp1  pt2=hp2  pt3=hp3  popup_f_axis=+Z
  Transform Align Axis Two Points : Suspension_Utilities/Transform Align Axis Two Points  hp_b=hp1  hp_t=hp2  popup_f_axis=-Z
  Translational Simscape Intf : Suspension_Utilities/Translational Simscape Intf  SystemSampleTime=-1  VariantActivationTime=update diagram  Latency=0  AutoFrameSizeCalculation=off
  Universal Two HP : Suspension_Utilities/Universal Two HP  popup_leftRight=Left  hp_f=hp_in_f_ua  hp_r=hp_in_r_ua
